simulink model "fluidDynamicSurface_th"  (R2018b)
settings: Solver=VariableStepAuto  StartTime=0.0  StopTime=0  RelTol=1e-3
values from neighbouring files (symbols this model uses):
  angVelBdy = [0 0 0]    [fluidDynamicSurface_ts.m]
  ctrlSurfDefl = 0    [fluidDynamicSurface_ts.m]
  velCMBdy = [0 0 0]    [fluidDynamicSurface_ts.m]
  velWindBdy = [0 0.1 0.0]    [fluidDynamicSurface_ts.m]
libraries: fluidDynamicSurface_cl x1
settings Model: Creator=mcobb  LastModifiedBy=mcobb

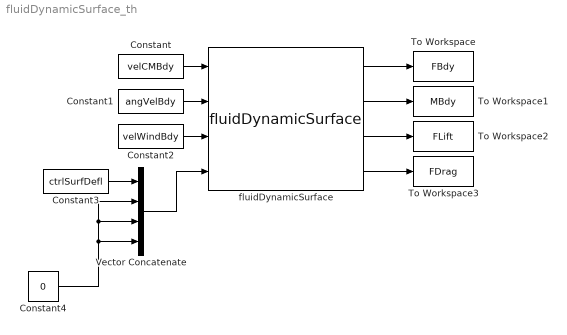
== system fluidDynamicSurface_th ==
  Constant : Constant  Value=velCMBdy
  Constant1 : Constant  Value=angVelBdy
  Constant2 : Constant  Value=velWindBdy
  Constant3 : Constant  Value=ctrlSurfDefl
  Constant4 : Constant  Value=0
  To Workspace : ToWorkspace  VariableName=FBdy  SaveFormat=Timeseries  SampleTime=-1
  To Workspace1 : ToWorkspace  VariableName=MBdy  SaveFormat=Timeseries  SampleTime=-1
  To Workspace2 : ToWorkspace  VariableName=FLift  SaveFormat=Timeseries  SampleTime=-1
  To Workspace3 : ToWorkspace  VariableName=FDrag  SaveFormat=Timeseries  SampleTime=-1
  Vector Concatenate : Concatenate  NumInputs=4
  fluidDynamicSurface : fluidDynamicSurface_cl/fluidDynamicSurface  aeroStruct=aeroSurf  fluidDensity=fluidDensity
  wires:
  fluidDynamicSurface/1 -> To Workspace/1
  Constant/1 -> fluidDynamicSurface/1
  Constant1/1 -> fluidDynamicSurface/2
  Constant2/1 -> fluidDynamicSurface/3
  Constant3/1 -> Vector Concatenate/1
  fluidDynamicSurface/3 -> To Workspace2/1
  fluidDynamicSurface/4 -> To Workspace3/1
  Vector Concatenate/1 -> fluidDynamicSurface/4
  Constant4/1 -> Vector Concatenate/4, Vector Concatenate/3, Vector Concatenate/2
  fluidDynamicSurface/2 -> To Workspace1/1
